simulink model "Multiplexer4x1"  (R2025b)
settings: Solver=VariableStepAuto  StartTime=0.0  StopTime=10.0  RelTol=1e-3
settings Model: Creator=jerin  LastModifiedBy=Johan

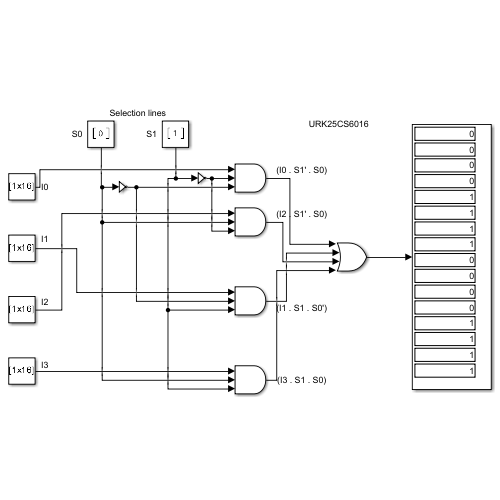
[thumbnail: Simulink's stored preview of the top-level diagram]
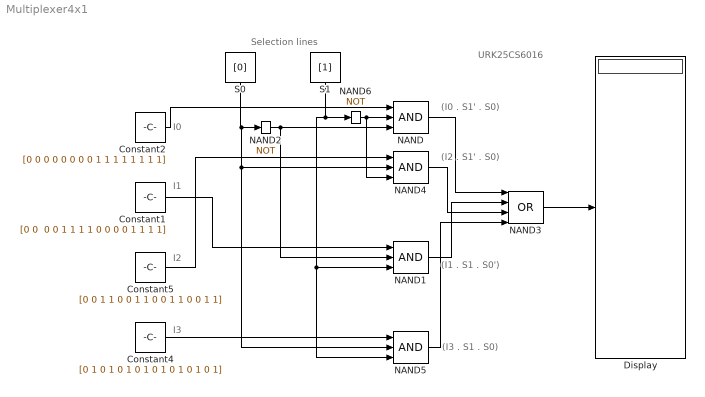
== system Multiplexer4x1 ==
  note: (I0 . S1' . S0)
  note: Selection lines
  note: I0
  note: URK25CS6016
  note: I1
  note: I3
  note: I2
  note: (I2 . S1' . S0)
  note: (I1 . S1 . S0')
  note: (I3 . S1 . S0)
  Constant1 : Constant  Value="[0 0  0 0 1 1 1 1 0 0 0 0 1 1 1 1]"
  Constant2 : Constant  Value=[0 0 0 0 0 0 0 0 1 1 1 1 1 1 1 1]
  Constant4 : Constant  Value=[0 1 0 1 0 1 0 1 0 1 0 1 0 1 0 1]
  Constant5 : Constant  Value=[0 0 1 1 0 0 1 1 0 0 1 1 0 0 1 1]
  Display : Display
  NAND{,1,4..5} (4 alike) : Logic  Inputs=3  IconShape=distinctive  AllPortsSameDT=off  OutDataTypeStr=boolean
  NAND2 : Logic  Operator=NOT  IconShape=distinctive  AllPortsSameDT=off  OutDataTypeStr=boolean
  NAND3 : Logic  Operator=OR  Inputs=4  IconShape=distinctive  AllPortsSameDT=off  OutDataTypeStr=boolean
  NAND6 : Logic  Operator=NOT  IconShape=distinctive  AllPortsSameDT=off  OutDataTypeStr=boolean
  S0 : Constant  Value=[0]
  S1 : Constant  Value=[1]
  wires:
  Constant2/1 -> NAND/1
  Constant1/1 -> NAND1/1
  NAND/1 -> NAND3/1
  NAND1/1 -> NAND3/2
  NAND3/1 -> Display/1
  Constant4/1 -> NAND5/1
  Constant5/1 -> NAND4/1
  NAND4/1 -> NAND3/3
  S1/1 -> NAND5/3, NAND1/3, NAND6/1
  S0/1 -> NAND2/1, NAND5/2, NAND4/2
  NAND2/1 -> NAND1/2, NAND/3
  NAND6/1 -> NAND4/3, NAND/2
  NAND5/1 -> NAND3/4
